simulink model "car_model"  (R2019b)
settings: Solver=ode23tb  StartTime=0.0  StopTime=60  RelTol=1e-3
InitFcn:
  | CommonVariables
  | Klqr5Velocities
values from neighbouring files (symbols this model uses):
  BattChrgMax = -80000    [CommonVariables.m]
  BattDischrgMax = 80000    [CommonVariables.m]
  BrkPrsMax = 5000000    [CommonVariables.m]
  ChrgLmt_bpt = [1 1 1 1 1 1 1 1 0.7 0.35 0]    [CommonVariables.m]
  DischrgLmt_bpt = [0 0.35 0.7 1 1 1 1 1 1 1 1]    [CommonVariables.m]
  disk_abore = 0.05    [CommonVariables.m]
  efficiency_table = [85 85 85 85 85 85 85 85 85 85 85 85 85 85 85;85 85 85 85 85 85 85 85 85 85 85 85 85 85 85;85 85 90 90 90 90 90 90 90 90 88 88 88 88 88;85 85 92 92 92 92 92 92 92 92 92 90 90 90 90;85 85 92 92 93 93 93 93 92 92 92 90 90 90 90;85 85 93 94 94 94 94 94 94 94 94 94 94 94 94;85 85 93 94 94 95 95 95 95 95 95 95 95 95 95;85 85 93 94 94 95 95 95 95 95 95 95 95 95 95;85 85 93 94 95 95 95 95 95 95 95 95 95  ...(+141 chars)    [CommonVariables.m]
  F0z = [2886 2907]    [CommonVariables.m]
  h = 0.134    [CommonVariables.m]
  m = 1200    [Klqr5Velocities.m]
  MotSpd = [0 1000 2000 2728.370453 3000 4000 5000 6000 7000 8000 9000 10000]    [CommonVariables.m]
  MotTrq = [280 280 280 280 254.6479089 190.9859317 152.7887454 127.3239545 109.1348181 95.49296586 84.88263632 76.39437268]    [CommonVariables.m]
  mu_kinetic = 0.35    [CommonVariables.m]
  Ndiff = 7.94    [CommonVariables.m]
  num_pads = 2    [CommonVariables.m]
  RegenBrkCutOff = [0 1]    [CommonVariables.m]
  RegenBrkSpd_bpt = [5 9]    [CommonVariables.m]
  Rm = 0.15    [CommonVariables.m]
  SOC_bpt = [0 10 20 30 40 50 60 70 80 90 100]    [CommonVariables.m]
  T_eff_bp = [0 20 40 60 80 100 120 140 160 180 200 220 240 260 280]    [CommonVariables.m]
  w_eff_bp = [0 1000 2000 2728.370453 3000 4000 5000 6000 7000 8000 9000 10000]    [CommonVariables.m]
undefined symbols (not defined in the file or in its folder): Disabled, DLCXref, DLCYref, Klqr1, Klqr2, Klqr3, Klqr4, Klqr5, Right, VEH
libraries: simulink x8, vehdynlibtire x8, vehdynlibsuspension x7, vehdynlibscenariocommon x5, autolibutils x4, sim3dlib x4, autolibmappedmotor x4, autolibshared x2, sharedtransform x2, vehdynlibviscommon x2, vehdynlibdriver x1, vehdynlibsteering x1
(part 1 of 7)
settings Model: SimulationMode=accelerator  OrderedModelArguments=off  Creator=davide  LastModifiedBy=alelu
settings SolverCC: ZeroCrossAlgorithm=Adaptive  AutoInsertRateTranBlk=on  InsertRTBMode=Never (minimum delay)
settings DebuggingCC: ArtificialAlgebraicLoopMsg=none  ModelReferenceExtraNoncontSigs=none
settings ModelReferenceCC: ModelReferenceMinAlgLoopOccurrences=on  PropagateSignalLabelsOutOfModel=off
settings SFSimCC: CustomCodeUndefinedFunction=UseInterfaceOnly

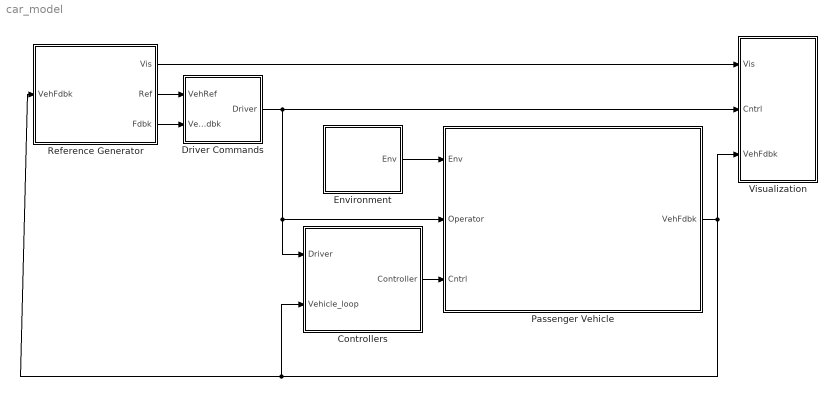
== system car_model ==
  Controllers : Subsystem
      mask Display: image('SystemControllers.png')
  Driver Commands : Subsystem  VariantControl=0  mask{driverType=Predictive Driver}
      mask prompts: driverType "Vehicle command mode"
      mask init:
      | [~]=vdynblksdrvrconfig(gcb)
      settings: AttributesFormatString=%<driverType>
      mask Help: eval('vdynblkshelp(''vdcrdriver'')');
      mask TypeOptions driverType: Longitudinal Driver | Predictive Driver | Open Loop
      mask Display: image('driverlatlong.png');
  Environment : Subsystem
      mask Display: disp('Environment')
  Passenger Vehicle : Subsystem
      mask Display: image('PassengerVehicle.png')
  Reference Generator : Subsystem  mask(Reference Generator){manType=Double Lane Change, manOverride=on, prevType=Double Lane Change, t_start=1, xdot_r=35, xdotUnit=mph, aMode=2, omega_hw=13.5, theta_max=90, t_stop=60, ay_max=.5, ay_stop=on, XGate=174.5, xStart=2, vehW=2, lattoff=VEH.InitialLatPosition, latRefbp=DLCXref, latRef=DLCYref, t_sweep=30, theta_hw=90, theta_hw_final=.7, steerF=.7, steerA=90, tdwell=.5, steerDir=off, R=100, turnDirMask=Right, cr_ay_max=0.5, cr_ay_stop=off, simTime=60, engine3D=Disabled, SceneDesc=Open surface, dt3D=.03, defaultPos=Recommended for scene, X_o=0, Y_o=0, Z_o=0, phi_o=0, theta_o=0, psi_o=0}
      mask prompts: manType "Maneuver"; manOverride "Use maneuver-specific driver, initial position, and scene"; t_start "Maneuver start time, t_start [s]:"; xdot_r "Longitudinal velocity reference, xdot_r:"; xdotUnit "Longitudinal entrance velocity setpoint units, xdotUnit []:"; omega_hw "Handwheel rate, omega_hw [deg/s]:"; theta_max "Maximum handwheel angle, theta_max [deg]:"; t_stop "Steering hold time after max angle reached, t_stop [s]:"; ay_max "Lateral acceleration threshold, ay_max [g]:"; ay_stop "Stop simulation at lateral acceleration threshold"; XGate "Inertial longitudinal position of gate entrance, XGate [m]:"; xStart "Distance after target speed to begin reference, x_start [m]:"; vehW "Vehicle width, vehW [m]:"; lattoff "Lateral offset, latoff [m]:"; latRefbp "Lateral reference position breakpoints [m]:"; latRef "Lateral reference data, latRef [m]:"; t_sweep "Swept time, t_sweep [s]:"; theta_hw "Steering amplitude, theta_hw [deg]"; theta_hw_final "Final frequency, theta_hw_final [Hz]:"; steerF "Steer frequency, steerF [Hz]:"; steerA "Steer amplitude, steerA [deg]:"; tdwell "Dwell time, tdwell [s]:"; steerDir "Change direction, steerDir"; R "Radius value, R [m]:"; turnDirMask "Turn direction"; cr_ay_max "Lateral acceleration threshold, ay_max [g]:"; cr_ay_stop "Stop simulation at lateral acceleration threshold"; simTime "Simulation time, simTime [s]:"; engine3D "3D Engine"; SceneDesc "Scene:"; dt3D "Engine frame rate, dt3D [s]:"; X_o "Initial longitudinal position, X_o [m]:"; Y_o "Initial lateral position, Y_o [m]:"; Z_o "Initial vertical position, Z_o [m]:"; phi_o "Initial roll angle, phi_o [rad]:"; theta_o "Initial pitch angle, theta_o [rad]:"; psi_o "Initial yaw angle, psi_o [rad]:"
      mask help: Set parameters to configure the maneuver, driver model, and 3D environment. To set the initial vehicle position and orientation, use the parameters on the 3D Engine tab.
      mask init:
      | set_param(gcb,'prevType',get_param(gcb,'manType'))
      settings: AttributesFormatString=%<manType>
      mask Help: eval('vdynblkshelp(''vdcrrefgen'')');
      mask TypeOptions manType: Double Lane Change | Increasing Steer | Swept Sine | Sine with Dwell | Constant Radius
      mask Callback manType:
      | [~]=vdynblksrefconfig(gcb,0);
      | [~]=vdynblksrefconfig(gcb,1);
      mask TypeOptions prevType: Double Lane Change | Increasing Steer | Swept Sine | Sine with Dwell | Constant Radius
      mask TypeOptions xdotUnit: Reference Generator/Double Lane Change/Double Lane Change/xdotUnit | Reference Generator/Constant Radius/xdotUnit | Reference Generator/Increasing Steer/Increasing Steer/xdotUnit | Reference Generator/Sine with Dwell/Sine With Dwell/xdotUnit | Reference Generator/Swept Sine/Swept Sine/xdotUnit
      mask TypeOptions omega_hw: Reference Generator/Increasing Steer/Increasing Steer/omega_hw
      mask TypeOptions theta_max: Reference Generator/Increasing Steer/Increasing Steer/theta_max
      mask TypeOptions t_stop: Reference Generator/Increasing Steer/Increasing Steer/t_stop
      mask TypeOptions ay_max: Reference Generator/Increasing Steer/Increasing Steer/ay_max
      mask TypeOptions ay_stop: Reference Generator/Increasing Steer/Increasing Steer/ay_stop
      mask Callback ay_stop:
      | if strcmp(get_param(gcb,'ay_stop'),'off')
      |     autoblksenableparameters(gcb, [], {'ay_max'},[],[],true);
      | else
      |     autoblksenableparameters(gcb,{'ay_max'},[],[],[],true);
      | end
      mask TypeOptions XGate: Reference Generator/Double Lane Change/Double Lane Change/XGate
      mask TypeOptions xStart: Reference Generator/Double Lane Change/Double Lane Change/xStart
      mask TypeOptions vehW: Reference Generator/Double Lane Change/Double Lane Change/vehW
      mask TypeOptions lattoff: Reference Generator/Double Lane Change/Double Lane Change/lattoff
      mask TypeOptions latRefbp: Reference Generator/Double Lane Change/Double Lane Change/latRefbp
      mask TypeOptions latRef: Reference Generator/Double Lane Change/Double Lane Change/latRef
      mask TypeOptions t_sweep: Reference Generator/Swept Sine/Swept Sine/t_sweep
      mask TypeOptions theta_hw: Reference Generator/Swept Sine/Swept Sine/theta_hw
      mask TypeOptions theta_hw_final: Reference Generator/Swept Sine/Swept Sine/theta_hw_final
      mask TypeOptions steerF: Reference Generator/Sine with Dwell/Sine With Dwell/steerF
      mask TypeOptions steerA: Reference Generator/Sine with Dwell/Sine With Dwell/steerA
      mask TypeOptions tdwell: Reference Generator/Sine with Dwell/Sine With Dwell/tdwell
      mask TypeOptions steerDir: Reference Generator/Sine with Dwell/Sine With Dwell/steerDir
      mask TypeOptions R: Reference Generator/Constant Radius/R
      mask TypeOptions turnDirMask: Reference Generator/Constant Radius/turnDirMask
      mask TypeOptions cr_ay_max: Reference Generator/Constant Radius/ay_max
      mask TypeOptions cr_ay_stop: Reference Generator/Constant Radius/ay_stop
      mask Callback cr_ay_stop:
      | if strcmp(get_param(gcb,'cr_ay_stop'),'off')
      |     autoblksenableparameters(gcb, [], {'cr_ay_max'},[],[],true);
      | else
      |     autoblksenableparameters(gcb,{'cr_ay_max'},[],[],[],true);
      | end
      mask TypeOptions engine3D: 3D Engine/engine3D
      mask TypeOptions SceneDesc: 3D Engine/SceneDesc
      mask Callback SceneDesc: [~] = vdynblks3Dsceneconfig(gcb);
      mask TypeOptions dt3D: 3D Engine/dt3D
      mask TypeOptions defaultPos: Recommended for scene | User-specified
      mask TypeOptions X_o: 3D Engine/X_o
      mask TypeOptions Y_o: 3D Engine/Y_o
      mask TypeOptions Z_o: 3D Engine/Z_o
      mask TypeOptions phi_o: 3D Engine/phi_o
      mask TypeOptions theta_o: 3D Engine/theta_o
      mask TypeOptions psi_o: 3D Engine/psi_o
      mask DialogControl modTab Prompt: Model
      mask DialogControl configGroup Prompt: Configuration
      mask DialogControl ISGroup Prompt: Increasing Steer
      mask DialogControl DLCGroup Prompt: Double Lane Change
      mask DialogControl SSGroup Prompt: Swept Sine
      mask DialogControl SDGroup Prompt: Sine with Dwell
      mask DialogControl CRGroup Prompt: Constant Radius
      mask DialogControl simUpdate Prompt: Set Model Simulation Time
      mask DialogControl simUpdate Callback: [~]=vdynblksrefconfig(gcb,2);
      mask DialogControl sim3DTab Prompt: 3D Engine
      mask DialogControl sim3DGroup Prompt: 3D Engine
      mask DialogControl posSetupDesc Prompt: To use these initial vehicle positions, first Apply the initial values and then click Update the model workspaces with the initial values.
      mask DialogControl setModelPos Prompt: Update model workspaces with initial values
      mask DialogControl setModelPos Callback: [~] = vdynblksmdlWSconfig(gcb);
      mask Display: image('vdbslibscen.png')
  Visualization : Subsystem
      mask Display: disp('Visualization')
  wires:
  Passenger Vehicle/1(VehFdbk) -> Controllers/2(Vehicle_loop), Reference Generator/1("VehFdbk "), Visualization/3(VehFdbk)
  Reference Generator/1(" Vis") -> Visualization/1(Vis)
  Reference Generator/2(" Ref") -> Driver Commands/1(VehRef)
  Controllers/1(Controller) -> Passenger Vehicle/3(Cntrl)
  Reference Generator/3(" Fdbk") -> Driver Commands/2(VehFdbk)
  Environment/1(Env) -> Passenger Vehicle/1(Env)
  Driver Commands/1(Driver) -> Passenger Vehicle/2(Operator), Controllers/1(Driver), Visualization/2(Cntrl)

== system car_model/Controllers ==
  Driver : Inport
  Vehicle_loop : Inport  Port=2
  Accel Pedal to Traction Wheel Torque Request : Subsystem
  Battery Management System : Subsystem
  Brake Pedal to Total Braking Pressure Request : Subsystem
  Bus Creator2 : BusCreator  Inputs=1
  Bus Creator3 : BusCreator  Inputs=3
  Bus Selector : BusSelector  OutputSignals=Body.r,Body.xdot,Body.ydot,Driveline.WhlAng,ElecFdbk.BattSoc,Driveline.EngSpd
  Bus Selector3 : BusSelector  OutputSignals=Steer,Accel,Brake
  Constant : Constant  Value=0
  Motor Torque Arbitration and Power Management : Subsystem
  Regen Braking Control : Subsystem  VariantControlMode=Label  Variant=on  VariantControl=(default)  LabelModeActiveChoice=Variant
  Controller : Outport  VectorParamsAs1DForOutWhenUnconnected=off
  wires:
  Driver/1 -> Bus Selector3/1
  Motor Torque Arbitration and Power Management/1(MotTrqCmdFinal) -> Bus Creator3/1  "acc"
  Bus Creator2/1 -> Bus Creator3/2  "Brake"
  Bus Creator3/1 -> Controller/1  "Controller"
  Battery Management System/1(BattPwrDischrgLmt) -> Motor Torque Arbitration and Power Management/3(BattPwrDisChrgLmt)  "BattPwrDischrgLmt"
  Regen Braking Control/1(" MotTrqCmdRegen") -> Motor Torque Arbitration and Power Management/6(MotTrqCmdRegen)  "MotTrqCmdRegen"
  [MotSpd] -> Motor Torque Arbitration and Power Management/5(MotSpd)
  Bus Selector/6 -> Regen Braking Control/2("VehSpd "), [MotSpd], Regen Braking Control/3("MotSpd ")  "<EngSpd>"
  Accel Pedal to Traction Wheel Torque Request/1(TrqCmd) -> Motor Torque Arbitration and Power Management/1(MotTrqCmdTrac)
  Battery Management System/2(BattPwrChrgLmt) -> Motor Torque Arbitration and Power Management/4("BattPwrChrgLmt ")  "BattPwrChrgLmt"
  Bus Selector3/3 -> Brake Pedal to Total Braking Pressure Request/1(DecelPdl)  "<Brake>"
  Regen Braking Control/2(" BrkCmd") -> Bus Creator2/1  "BrkCmd"
  Constant/1 -> Brake Pedal to Total Braking Pressure Request/2(Park)
  [MotSpd] -> Accel Pedal to Traction Wheel Torque Request/6(MotSpd)
  Bus Selector/5 -> Battery Management System/1(SOC), Regen Braking Control/1("BattSoc ")  "<BattSoc>"
  Brake Pedal to Total Braking Pressure Request/1(BrkPrsReq) -> Regen Braking Control/4("BrkPrsReq ")
  [AccelPdl] -> Motor Torque Arbitration and Power Management/2(AccelPdl)
  Bus Selector3/2 -> Accel Pedal to Traction Wheel Torque Request/1(AccelPdl), [AccelPdl]  "<Accel>"
  Vehicle_loop/1 -> Bus Selector/1
  Bus Selector/4 -> Accel Pedal to Traction Wheel Torque Request/2(WhlAng)  "<WhlAng>"
  Bus Selector/1 -> Accel Pedal to Traction Wheel Torque Request/5(YawRate)  "<r>"
  Bus Selector/2 -> Accel Pedal to Traction Wheel Torque Request/3(xdot)  "<xdot>"
  Bus Selector/3 -> Accel Pedal to Traction Wheel Torque Request/4(ydot)  "<ydot>"

== system car_model/Driver Commands ==
  VehRef : Inport
  VehFdbk : Inport  Port=2
  AccelGround : Ground
  BrakeGround : Ground
  Driver Commands : Subsystem  VariantControlMode=Label  Variant=on  VariantControl=Variant1  LabelModeActiveChoice=1  AllowZeroVariantControls=on
  GearGround : Ground
  SteerGround : Ground
  Driver : Outport  VectorParamsAs1DForOutWhenUnconnected=off
  wires:
  VehRef/1 -> Driver Commands/1(VehRef)
  VehFdbk/1 -> Driver Commands/2(VehFdbk)
  Driver Commands/1(" Driver") -> Driver/1
  SteerGround/1 -> Driver Commands/3(SteerCmd)
  AccelGround/1 -> Driver Commands/4(Accel)
  BrakeGround/1 -> Driver Commands/5(Brake)
  GearGround/1 -> Driver Commands/6(Gear)

== system car_model/Environment ==
  Bus Creator1 : BusCreator  Inputs=4
  Constant3 : Constant  Value=0
  Constant4 : Constant  Value=0
  Constant5 : Constant  Value=0
  Constant6 : Constant  Value=300
  Constant7 : Constant  Value=101325
  Friction : Constant  Value=ones(4,1).*1
  Ground Feedback : Subsystem  VariantControlMode=Label  Variant=on  LabelModeActiveChoice=0
  Vector Concatenate : Concatenate  NumInputs=3
  Env : Outport  VectorParamsAs1DForOutWhenUnconnected=off
  wires:
  Constant5/1 -> Vector Concatenate/3  "Z"
  Vector Concatenate/1 -> Bus Creator1/3  "Wind"
  Constant3/1 -> Vector Concatenate/1  "X"
  Constant4/1 -> Vector Concatenate/2  "Y"
  Ground Feedback/1(Ground) -> Bus Creator1/4  "Gnd"
  Bus Creator1/1 -> Env/1
  Friction/1 -> Ground Feedback/1(Friction)
  Constant6/1 -> Bus Creator1/1  "Temp"
  Constant7/1 -> Bus Creator1/2  "Baro"

== system car_model/Passenger Vehicle ==
  Env : Inport
  Operator : Inport  Port=2
  Cntrl : Inport  Port=3
  Bus Creator2 : BusCreator  Inputs=4
  Subsystem : Subsystem
  Subsystem1 : Subsystem
  Subsystem2 : Subsystem
  Subsystem4 : Subsystem
  Subsystem5 : Subsystem
  Subsystem6 : Subsystem
  VehFdbk : Outport  VectorParamsAs1DForOutWhenUnconnected=off
  wires:
  Bus Creator2/1 -> VehFdbk/1
  Env/1 -> Subsystem2/4(Env), Subsystem/1(Env)
  Subsystem1/1(Driveline) -> [Driveline], Bus Creator2/1  "Driveline"
  Subsystem5/1(WhlAng) -> Subsystem1/1(WhlAng)
  Operator/1 -> Subsystem2/2(SteerCmd)
  Cntrl/1 -> Subsystem2/1(Cntrl)
  Subsystem2/1(Steer) -> Subsystem5/1(SteerHWCmd)
  Subsystem2/2(brake) -> Subsystem5/2(BrkPrsCmd)
  Subsystem4/2(Wheels) -> Bus Creator2/4, [Wheels]  "Wheels"
  [Driveline] -> Subsystem/2(Driveline)
  [Wheels] -> Subsystem2/3(Wheels)
  Subsystem6/15(dzWheel) -> Subsystem4/15(dzWheel)
  Subsystem6/3(CgXYZdot) -> Subsystem4/3(CgXYZdot)
  Subsystem6/1(Cgxyzdot) -> Subsystem4/1(Cgxyzdot)
  Subsystem6/5(pqr) -> Subsystem4/5(pqr)
  Subsystem6/14(YWheel) -> Subsystem4/14(YWheel)
  Subsystem6/7(Beta) -> Subsystem4/7(Beta)
  Subsystem6/6(Cgaxyz) -> Subsystem4/6(Cgaxyz)
  Subsystem6/8(GeomXYZ) -> Subsystem4/8(GeomXYZ)
  Subsystem6/4(angles) -> Subsystem4/4(angles)
  Subsystem6/11(kappa) -> Subsystem4/11(kappa)
  Subsystem6/13(XWheel) -> Subsystem4/13(XWheel)
  Subsystem6/2(CgXYZ) -> Subsystem4/2(CgXYZ)
  Subsystem6/9(GeomXYZdot) -> Subsystem4/9(GeomXYZdot)
  Subsystem6/10(omega) -> Subsystem4/10(omega)
  Subsystem6/12(alpha) -> Subsystem4/12(alpha)
  Subsystem5/2(BrkPrs) -> Subsystem1/2(BrkPrs)
  Subsystem5/5(BattSoc) -> Subsystem1/5(BattSoc)
  Subsystem5/6(BattPwr) -> Subsystem1/6(BattPwr)
  Subsystem5/7(BattCrnt) -> Subsystem1/7(BattCrnt)
  Subsystem2/4(acc) -> Subsystem5/4("acc ")
  Subsystem5/3(AxlTrq) -> Subsystem1/3(AxlTrq)
  Subsystem5/4(Motor_speed) -> Subsystem1/4(EngSpd)
  Subsystem2/5(amb_temp) -> Subsystem5/5(AmbTmp)
  Subsystem2/3(omega) -> Subsystem5/3(speed_wheel)
  Subsystem1/2(ElecFdbk) -> Bus Creator2/2  "ElecFdbk"
  Subsystem4/1(Chassis) -> Bus Creator2/3  "Body"
  Subsystem/1(Wind) -> Subsystem6/1(WindXYZ)
  Subsystem/2(Gnd) -> Subsystem6/2(Ground)
  Subsystem/3(mu) -> Subsystem6/3(Friction)
  Subsystem/4(WhlAng) -> Subsystem6/4(WheelAngle)
  Subsystem/5(AxleTrq) -> Subsystem6/5(AxleTrq)
  Subsystem/6(BrkPrs) -> Subsystem6/6(BrkPrs)

== system car_model/Reference Generator ==
  "VehFdbk " : Inport
  3D Engine : Subsystem  VariantControlMode=Label  Variant=on  LabelModeActiveChoice=0  mask(3D Engine){engine3D=Disabled, SceneDesc=Open surface, dt3D=dt3D, defaultPos=User-specified, X_o=X_o, Y_o=Y_o, Z_o=Z_o, phi_o=phi_o, theta_o=theta_o, psi_o=psi_o}
      mask prompts: engine3D "3D Engine"; SceneDesc "Scene:"; dt3D "Engine frame rate, dt3D [s]:"; X_o "Initial longitudinal position, X_o [m]:"; Y_o "Initial lateral position, Y_o [m]:"; Z_o "Initial vertical position, Z_o [m]:"; phi_o "Initial roll angle, phi_o [rad]:"; theta_o "Initial pitch angle, theta_o [rad]:"; psi_o "Initial yaw angle, psi_o [rad]:"
      mask help: This subsystem contains the interface blocks which permit the display of the vehicle in the 3D virtual environment. Enable it to view the simulation progress, disable it to inhibit the display.
      mask init:
      | switch get_param(gcb,'engine3D')
      |     case 'Disabled'
      |         set_param(gcb,'OverrideUsingVariant','0')
      |         try
      |             set_param([bdroot '/Environment/Ground Feedback'],'OverrideUsingVariant','0')
      |         catch
      |             disp('Warning: No ground feedback sensor not set')
      |         end
      |     case 'Enabled'
      |         set_param(gcb,'OverrideUsingVariant','1')
      |         try
      |             set_param([bdroot '/Environment/Ground Feedback'],'OverrideUsingVariant','1')
      |         catch
      |             disp('Warning: No ground feedback sensor not set')
      |         end
      |     otherwise
      |         set_param(gcb,'OverrideUsingVariant','0')
      | end
      settings: AttributesFormatString=|
      | %<SceneDesc>
      | %<engine3D>
      mask Help: eval('vdynblkshelp(''vdynblks3dengine'')');
      mask TypeOptions engine3D: Enabled | Disabled
      mask Callback engine3D:
      | switch get_param(gcb,'engine3D')
      |     case 'Disabled'
      |         set_param(gcb,'OverrideUsingVariant','0')
      |     case 'Enabled'
      |        set_param(gcb,'OverrideUsingVariant','1')
      |     otherwise
      |        set_param(gcb,'OverrideUsingVariant','0')
      | end
      mask TypeOptions SceneDesc:
      | 3D Engine/Simulation 3D Engine
      | 1/SceneDesc
      mask Callback SceneDesc: [~] = vdynblks3Dsceneconfig(gcb);
      mask TypeOptions defaultPos: Recommended for scene | User-specified
      mask DialogControl engineConfig Prompt: 3D Engine Settings
      mask DialogControl posSetup Prompt: Initial vehicle position
      mask DialogControl posSetupDesc Prompt: To use these initial vehicle positions, first Apply the initial values and then click Update the model workspaces with the initial values.
      mask DialogControl setModelPos Prompt: Update model workspaces with initial values
      mask DialogControl setModelPos Callback: [~] = vdynblksmdlWSconfig(gcb);
      mask Display: disp('3D Engine')
  Reference Generator : Subsystem  VariantControlMode=Label  Variant=on  VariantControl=Variant1  LabelModeActiveChoice=4
  " Vis" : Outport  VectorParamsAs1DForOutWhenUnconnected=off
  " Ref" : Outport  Port=2  VectorParamsAs1DForOutWhenUnconnected=off
  " Fdbk" : Outport  Port=3  VectorParamsAs1DForOutWhenUnconnected=off
  wires:
  "VehFdbk "/1 -> 3D Engine/1(VehFdbk), Reference Generator/1("VehFdbk ")
  Reference Generator/1(" Vis") -> " Vis"/1
  Reference Generator/2(" Ref") -> " Ref"/1
  Reference Generator/3(" Fdbk") -> " Fdbk"/1

== system car_model/Visualization ==
  note: Vehicle Response
  note: Driver Commands
  Vis : Inport
  Cntrl : Inport  Port=2
  VehFdbk : Inport  Port=3
  Acceleration Cmd : LinearGaugeBlock  LabelPosition=Hide  ScaleMax=1  TickInterval=0.20000000000000001
  Brake Cmd : LinearGaugeBlock  LabelPosition=Hide  ScaleMax=1  TickInterval=0.20000000000000001
  Bus Selector : BusSelector  OutputSignals=Body.xdot,Body.ay
  Bus Selector2 : BusSelector  OutputSignals=Accel,Brake,Steer
  Engine Tach [rpm] : CircularGaugeBlock  LabelPosition=Hide  ScaleMax=8000  TickInterval=1000
  Handwheel Angle [deg] : SemiCircularGaugeBlock  LabelPosition=Hide  ScaleMin=-300  ScaleMax=300  TickInterval=60
  ISO 15037-1:2006 : Subsystem  StopFcn=|  VariantControlMode=Label  Variant=on  LabelModeActiveChoice=0  mask(ISO 15037-1:2006){Measurement=Disabled}
      | switch get_param(gcb,'Measurement')
      |     case 'Enabled'
      |        p=slproject.getCurrentProject;
      |        projectRoot=p.RootFolder;
      |        SySFolder=fullfile(projectRoot, 'System');
      |        Simulink.sdi.loadView([SySFolder filesep 'ISO15037_1_2006E.mldatx']);
      |        Simulink.sdi.view;
      | end
      mask prompts: Measurement "ISO Measurements"
      mask help: Enables display of ISO 15037-1:2006 standard measurement signals in the Simulation Data Inspector.
      mask init:
      | switch get_param(gcb,'Measurement')
      |     case 'Disabled'
      |         set_param(gcb,'OverrideUsingVariant','0')
      |     case 'Enabled'
      |        set_param(gcb,'OverrideUsingVariant','1')
      |     otherwise
      |        set_param(gcb,'OverrideUsingVariant','0')
      | end
      settings: AttributesFormatString=%<Measurement>
      mask Help: eval('vdynblkshelp(''iso15037'')');
      mask TypeOptions Measurement: Enabled | Disabled
      mask Callback Measurement:
      | switch get_param(gcb,'Measurement')
      |     case 'Disabled'
      |         set_param(gcb,'OverrideUsingVariant','0')
      |     case 'Enabled'
      |        set_param(gcb,'OverrideUsingVariant','1')
      |     otherwise
      |        set_param(gcb,'OverrideUsingVariant','0')
      | end
      mask Display: disp('ISO 15037-1:2006')
  Lateral Acceleration [g] : SemiCircularGaugeBlock  LabelPosition=Hide  ScaleMin=-1  ScaleMax=1  TickInterval=0.5
  Rate Transition1 : RateTransition  Deterministic=off  OutPortSampleTime=.1
  Rate Transition2 : RateTransition  Deterministic=off  OutPortSampleTime=.1
  Scope Type : Subsystem  VariantControlMode=Label  Variant=on  VariantControl=Variant1  LabelModeActiveChoice=2
  Signal Specification : SignalSpecification  Unit=deg
  Signal Specification1 : SignalSpecification  Unit=mph
  Speed [mph] : CircularGaugeBlock  LabelPosition=Hide  TickInterval=10
  Steer vs Ay : simulink/Sinks/XY Graph  Commented=on  xmin=-300  xmax=300  ymin=-1.5  ymax=1.5  st=.1
  "Steer, Velocity, Lat Accel" : Scope  NumInputPorts=3
  Terminator : Terminator
  Terminator1 : Terminator
  Terminator2 : Terminator
  Unit Conversion1 : UnitConversion
  Unit Conversion2 : UnitConversion
  Vehicle XY Plotter : Subsystem  VariantControlMode=Label  Variant=on  VariantControl=Variant1  LabelModeActiveChoice=1
  wires:
  Signal Specification/1 -> Rate Transition1/1, "Steer, Velocity, Lat Accel"/1  "SteerAngle"
  Bus Selector/2 -> "Steer, Velocity, Lat Accel"/3, Rate Transition2/1  "<ay>"
  Bus Selector/1 -> "Steer, Velocity, Lat Accel"/2, Unit Conversion1/1  "<xdot>"
  Unit Conversion2/1 -> Signal Specification/1
  Unit Conversion1/1 -> Signal Specification1/1
  Signal Specification1/1 -> Terminator/1  "xdot_mph"
  Bus Selector2/3 -> Unit Conversion2/1  "<Steer>"
  Rate Transition1/1 -> Steer vs Ay/1
  Rate Transition2/1 -> Steer vs Ay/2
  Bus Selector2/1 -> Terminator1/1  "<Accel>"
  Bus Selector2/2 -> Terminator2/1  "<Brake>"
  VehFdbk/1 -> ISO 15037-1:2006/1(VehFdbk), Scope Type/1("VehFdbk "), Vehicle XY Plotter/1("VehFdbk "), Bus Selector/1  "VehFdbk"
  Cntrl/1 -> ISO 15037-1:2006/2(Cntrl), Scope Type/2(Cntrl), Bus Selector2/1
  Vis/1 -> Scope Type/3("Vis ")
  Scope Type/1(" Ref") -> Vehicle XY Plotter/2("Ref ")

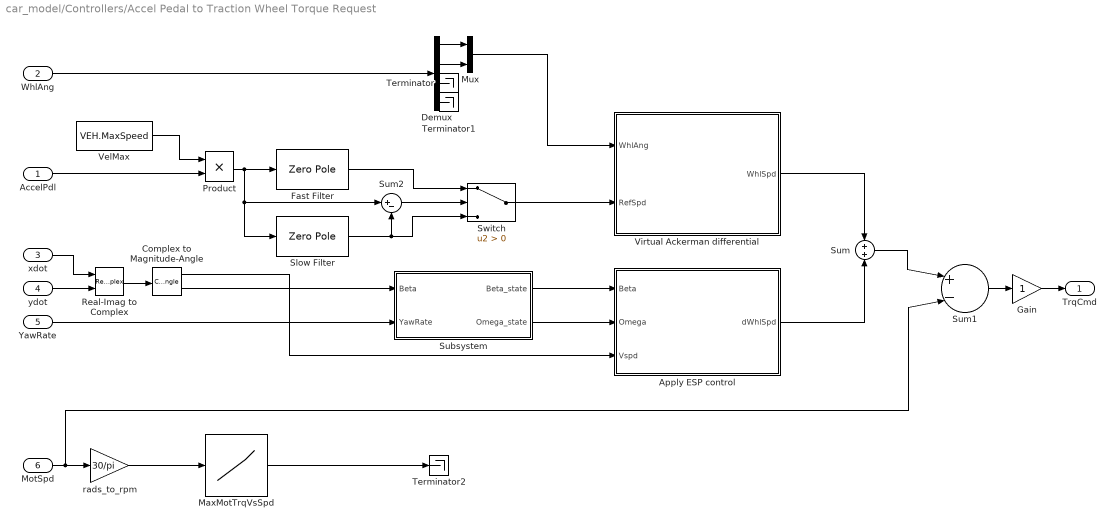
== system car_model/Controllers/Accel Pedal to Traction Wheel Torque Request ==
  AccelPdl : Inport
  WhlAng : Inport  Port=2
  xdot : Inport  Port=3
  ydot : Inport  Port=4
  YawRate : Inport  Port=5
  MotSpd : Inport  Port=6
  Apply ESP control : Subsystem
  Complex to Magnitude-Angle : ComplexToMagnitudeAngle
  Demux : Demux
  Fast Filter : ZeroPole  Zeros=[]  Poles=[-20]
  Gain : Gain
  MaxMotTrqVsSpd : Lookup_n-D  NumberOfTableDimensions=1  BreakpointsForDimension1=MotSpd  Table=MotTrq  ExtrapMethod=Clip  UseLastTableValue=on  InternalRulePriority=Speed  OutDataTypeStr=Inherit: Inherit from 'Table data'  RndMeth=Simplest  InputSameDT=on
  Mux : Mux  Inputs=2
  Product : Product
  Real-Imag to Complex : RealImagToComplex
  Slow Filter : ZeroPole  Zeros=[]  Poles=[-2]
  Subsystem : Subsystem
  Sum : Sum  Inputs=+|+
  Sum1 : Sum  Inputs=|+-|
  Sum2 : Sum  Inputs=|+-
  Switch : Switch  Criteria=u2 > Threshold
  Terminator : Terminator
  Terminator1 : Terminator
  Terminator2 : Terminator
  VelMax : Constant  Value=VEH.MaxSpeed
  Virtual Ackerman differential : Subsystem
  rads_to_rpm : Gain  Gain=30/pi
  TrqCmd : Outport  VectorParamsAs1DForOutWhenUnconnected=off
  wires:
  MaxMotTrqVsSpd/1 -> Terminator2/1
  MotSpd/1 -> Sum1/2, rads_to_rpm/1
  rads_to_rpm/1 -> MaxMotTrqVsSpd/1
  Subsystem/1(Beta_state) -> Apply ESP control/1(Beta)
  Subsystem/2(Omega_state) -> Apply ESP control/2(Omega)
  Real-Imag to Complex/1 -> Complex to Magnitude-Angle/1
  xdot/1 -> Real-Imag to Complex/1
  ydot/1 -> Real-Imag to Complex/2
  Complex to Magnitude-Angle/1 -> Apply ESP control/3(Vspd)
  Complex to Magnitude-Angle/2 -> Subsystem/1(Beta)
  YawRate/1 -> Subsystem/2(YawRate)
  Virtual Ackerman differential/1(WhlSpd) -> Sum/1
  Apply ESP control/1(dWhlSpd) -> Sum/2
  Sum/1 -> Sum1/1
  VelMax/1 -> Product/1
  AccelPdl/1 -> Product/2
  Product/1 -> Fast Filter/1, Slow Filter/1, Sum2/1
  Fast Filter/1 -> Switch/1
  Sum1/1 -> Gain/1
  Gain/1 -> TrqCmd/1
  Demux/1 -> Mux/1
  Demux/2 -> Mux/2
  WhlAng/1 -> Demux/1
  Mux/1 -> Virtual Ackerman differential/1(WhlAng)
  Sum2/1 -> Switch/2
  Slow Filter/1 -> Switch/3, Sum2/2
  Switch/1 -> Virtual Ackerman differential/2(RefSpd)

== system car_model/Controllers/Battery Management System ==
  note: Behaviorial BMS System. Limits battery charge / discharge power based on SOC.
      |
      | Charge/Discharge Limits and curves can be adjusted if using a larger battery pack
      | or motor power is changed.
  SOC : Inport
  ChrgLmt : Lookup_n-D  NumberOfTableDimensions=1  BreakpointsForDimension1=SOC_bpt  Table=ChrgLmt_bpt  ExtrapMethod=Clip  UseLastTableValue=on  InternalRulePriority=Speed  RndMeth=Simplest  InputSameDT=on
  DischrgLmt : Lookup_n-D  NumberOfTableDimensions=1  BreakpointsForDimension1=SOC_bpt  Table=DischrgLmt_bpt  ExtrapMethod=Clip  UseLastTableValue=on  InternalRulePriority=Speed  RndMeth=Simplest  InputSameDT=on
  MaxChrg : Constant  Value=BattChrgMax
  MaxDischrg : Constant  Value=BattDischrgMax
  Product : Product
  Product1 : Product
  BattPwrDischrgLmt : Outport  VectorParamsAs1DForOutWhenUnconnected=off
  BattPwrChrgLmt : Outport  Port=2  VectorParamsAs1DForOutWhenUnconnected=off
  wires:
  SOC/1 -> DischrgLmt/1, ChrgLmt/1
  MaxChrg/1 -> Product1/2
  MaxDischrg/1 -> Product/2
  Product/1 -> BattPwrDischrgLmt/1
  Product1/1 -> BattPwrChrgLmt/1
  ChrgLmt/1 -> Product1/1
  DischrgLmt/1 -> Product/1

== system car_model/Controllers/Brake Pedal to Total Braking Pressure Request ==
  note: Converts Brake Pedal Position to Brake Pressure Request
  DecelPdl : Inport
  Park : Inport  Port=2
  Constant : Constant  Value=BrkPrsMax
  Constant1 : Constant
  Product1 : Product
  Switch : Switch  Criteria=u2 > Threshold
  BrkPrsReq : Outport  VectorParamsAs1DForOutWhenUnconnected=off
  wires:
  Constant/1 -> Product1/2
  Switch/1 -> Product1/1
  DecelPdl/1 -> Switch/3
  Constant1/1 -> Switch/1
  Product1/1 -> BrkPrsReq/1
  Park/1 -> Switch/2

== system car_model/Controllers/Motor Torque Arbitration and Power Management ==
  MotTrqCmdTrac : Inport
  AccelPdl : Inport  Port=2
  BattPwrDisChrgLmt : Inport  Port=3
  "BattPwrChrgLmt " : Inport  Port=4
  MotSpd : Inport  Port=5
  MotTrqCmdRegen : Inport  Port=6
  Accel Decel Switch : Switch  Criteria=u2 > Threshold
  Compare To Constant : simulink/Logic and Bit Operations/Compare To Constant  relop=>  const=0  OutDataTypeStr=boolean
  Power Management : Subsystem
  MotTrqCmdFinal : Outport  VectorParamsAs1DForOutWhenUnconnected=off
  wires:
  AccelPdl/1 -> Compare To Constant/1
  MotTrqCmdRegen/1 -> Accel Decel Switch/3
  MotTrqCmdTrac/1 -> Accel Decel Switch/1
  Power Management/1(MotTrqCmdFinal) -> MotTrqCmdFinal/1
  Accel Decel Switch/1 -> Power Management/4(MotTrqCmd)
  BattPwrDisChrgLmt/1 -> Power Management/1(BattPwrDischrgLmt)
  "BattPwrChrgLmt "/1 -> Power Management/2(BattPwrChrgLmt)
  MotSpd/1 -> Power Management/3(MotSpd)
  Compare To Constant/1 -> Accel Decel Switch/2

== system car_model/Controllers/Regen Braking Control ==
  "BattSoc " : Inport
  "VehSpd " : Inport  Port=2
  "MotSpd " : Inport  Port=3
  "BrkPrsReq " : Inport  Port=4
  Parallel Regen Braking : Subsystem  InitFcn=%[~]=autosharedicon('autolibutils',gcb,0);  VariantControl=(default)
  Series Regen Braking : Subsystem  InitFcn=%[~]=autosharedicon('autolibutils',gcb,0);  VariantControl=Variant
  " MotTrqCmdRegen" : Outport  VectorParamsAs1DForOutWhenUnconnected=off
  " BrkCmd" : Outport  Port=2  VectorParamsAs1DForOutWhenUnconnected=off

== system car_model/Driver Commands/Driver Commands ==
  VehRef : Inport
  VehFdbk : Inport  Port=2
  SteerCmd : Inport  Port=3
  Accel : Inport  Port=4
  Brake : Inport  Port=5
  Gear : Inport  Port=6
  Longitudinal Driver : Subsystem  VariantControl=0
  Open Loop Constant Radius : Subsystem  VariantControl=2
  Predictive Driver : Subsystem  VariantControl=1
  " Driver" : Outport  VectorParamsAs1DForOutWhenUnconnected=off

== system car_model/Environment/Ground Feedback ==
  note: 1) Add Subsystem or Model blocks as valid variant choices.
      | 2) You cannot connect blocks at this level. At simulation, connectivity is automatically
      | determined, based on the active variant and port name matching.
  Friction : Inport
  3D Engine : Subsystem  VariantControl=1
  Constant : Subsystem  VariantControl=0
  Ground : Outport  VectorParamsAs1DForOutWhenUnconnected=off

== system car_model/Passenger Vehicle/Subsystem ==
  Env : Inport
  Driveline : Inport  Port=2
  Bus Selector1 : BusSelector  OutputSignals=Gnd.z.G_FL_z,Gnd.z.G_FR_z,Gnd.z.G_RL_z,Gnd.z.G_RR_z
  Bus Selector2 : BusSelector  OutputSignals=Wind
  Bus Selector3 : BusSelector  OutputSignals=Gnd.mu.mu_FL,Gnd.mu.mu_FR,Gnd.mu.mu_RL,Gnd.mu.mu_RR
  Bus Selector4 : BusSelector  OutputSignals=WhlAng,AxlTrq,BrkPrs
  Vector Concatenate : Concatenate  NumInputs=4
  Vector Concatenate1 : Concatenate  NumInputs=4
  Wind : Outport  VectorParamsAs1DForOutWhenUnconnected=off
  Gnd : Outport  Port=2  VectorParamsAs1DForOutWhenUnconnected=off
  mu : Outport  Port=3  VectorParamsAs1DForOutWhenUnconnected=off
  WhlAng : Outport  Port=4  VectorParamsAs1DForOutWhenUnconnected=off
  AxleTrq : Outport  Port=5  VectorParamsAs1DForOutWhenUnconnected=off
  BrkPrs : Outport  Port=6  VectorParamsAs1DForOutWhenUnconnected=off
  wires:
  Env/1 -> Bus Selector3/1, Bus Selector1/1, Bus Selector2/1
  Bus Selector2/1 -> Wind/1  "<Wind>"
  Bus Selector3/1 -> Vector Concatenate/1  "<mu_FL>"
  Bus Selector3/2 -> Vector Concatenate/2  "<mu_FR>"
  Bus Selector3/3 -> Vector Concatenate/3  "<mu_RL>"
  Bus Selector3/4 -> Vector Concatenate/4  "<mu_RR>"
  Vector Concatenate/1 -> mu/1
  Bus Selector1/1 -> Vector Concatenate1/1  "<G_FL_z>"
  Bus Selector1/2 -> Vector Concatenate1/2  "<G_FR_z>"
  Bus Selector1/3 -> Vector Concatenate1/3  "<G_RL_z>"
  Bus Selector1/4 -> Vector Concatenate1/4  "<G_RR_z>"
  Vector Concatenate1/1 -> Gnd/1
  Driveline/1 -> Bus Selector4/1
  Bus Selector4/2 -> AxleTrq/1  "<AxlTrq>"
  Bus Selector4/1 -> WhlAng/1  "<WhlAng>"
  Bus Selector4/3 -> BrkPrs/1  "<BrkPrs>"

== system car_model/Passenger Vehicle/Subsystem1 ==
  WhlAng : Inport
  BrkPrs : Inport  Port=2
  AxlTrq : Inport  Port=3
  EngSpd : Inport  Port=4
  BattSoc : Inport  Port=5
  BattPwr : Inport  Port=6
  BattCrnt : Inport  Port=7
  Bus Creator1 : BusCreator  Inputs=4
  Bus Creator3 : BusCreator  Inputs=4
  Driveline : Outport  VectorParamsAs1DForOutWhenUnconnected=off
  ElecFdbk : Outport  Port=2  VectorParamsAs1DForOutWhenUnconnected=off
  wires:
  Bus Creator1/1 -> Driveline/1  "Driveline"
  AxlTrq/1 -> Bus Creator1/2, Bus Creator3/4  "AxlTrq"
  WhlAng/1 -> Bus Creator1/1  "WhlAng"
  EngSpd/1 -> Bus Creator1/4  "EngSpd"
  BrkPrs/1 -> Bus Creator1/3  "BrkPrs"
  BattCrnt/1 -> Bus Creator3/3
  BattPwr/1 -> Bus Creator3/2
  BattSoc/1 -> Bus Creator3/1
  Bus Creator3/1 -> ElecFdbk/1  "ElecFdbk"

== system car_model/Passenger Vehicle/Subsystem2 ==
  Cntrl : Inport
  SteerCmd : Inport  Port=2
  Wheels : Inport  Port=3
  Env : Inport  Port=4
  Bus Selector1 : BusSelector  OutputSignals=Steer
  Bus Selector2 : BusSelector  OutputSignals=omega
  Bus Selector3 : BusSelector  OutputSignals=Brake,acc
  Bus Selector4 : BusSelector  OutputSignals=Temp
  Steer : Outport  VectorParamsAs1DForOutWhenUnconnected=off
  brake : Outport  Port=2  VectorParamsAs1DForOutWhenUnconnected=off
  omega : Outport  Port=3  VectorParamsAs1DForOutWhenUnconnected=off
  acc : Outport  Port=4  VectorParamsAs1DForOutWhenUnconnected=off
  amb_temp : Outport  Port=5  VectorParamsAs1DForOutWhenUnconnected=off
  wires:
  Cntrl/1 -> Bus Selector3/1
  SteerCmd/1 -> Bus Selector1/1
  Wheels/1 -> Bus Selector2/1
  Bus Selector2/1 -> omega/1  "<omega>"
  Bus Selector3/1 -> brake/1  "<Brake>"
  Bus Selector1/1 -> Steer/1  "<Steer>"
  Bus Selector3/2 -> acc/1  "<acc>"
  Bus Selector4/1 -> amb_temp/1  "<Temp>"
  Env/1 -> Bus Selector4/1

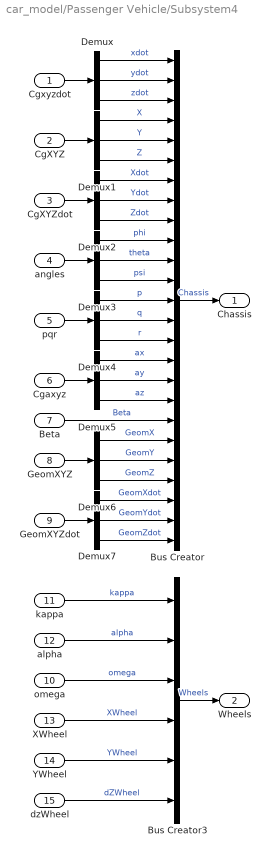
== system car_model/Passenger Vehicle/Subsystem4 ==
  Cgxyzdot : Inport
  CgXYZ : Inport  Port=2
  CgXYZdot : Inport  Port=3
  angles : Inport  Port=4
  pqr : Inport  Port=5
  Cgaxyz : Inport  Port=6
  Beta : Inport  Port=7
  GeomXYZ : Inport  Port=8
  GeomXYZdot : Inport  Port=9
  omega : Inport  Port=10
  kappa : Inport  Port=11
  alpha : Inport  Port=12
  XWheel : Inport  Port=13
  YWheel : Inport  Port=14
  dzWheel : Inport  Port=15
  Bus Creator : BusCreator  Inputs=25
  Bus Creator3 : BusCreator  Inputs=6
  Demux{,1..7} (8 alike) : Demux  Outputs=3
  Chassis : Outport  VectorParamsAs1DForOutWhenUnconnected=off
  Wheels : Outport  Port=2  VectorParamsAs1DForOutWhenUnconnected=off
  wires:
  Bus Creator/1 -> Chassis/1  "Chassis"
  omega/1 -> Bus Creator3/3  "omega"
  dzWheel/1 -> Bus Creator3/6  "dZWheel"
  kappa/1 -> Bus Creator3/1  "kappa"
  Bus Creator3/1 -> Wheels/1  "Wheels"
  YWheel/1 -> Bus Creator3/5  "YWheel"
  XWheel/1 -> Bus Creator3/4  "XWheel"
  alpha/1 -> Bus Creator3/2  "alpha"
  Cgxyzdot/1 -> Demux/1
  CgXYZ/1 -> Demux1/1
  CgXYZdot/1 -> Demux2/1
  angles/1 -> Demux3/1
  pqr/1 -> Demux4/1
  Cgaxyz/1 -> Demux5/1
  GeomXYZdot/1 -> Demux7/1
  GeomXYZ/1 -> Demux6/1
  Demux/1 -> Bus Creator/1  "xdot"
  Demux/2 -> Bus Creator/2  "ydot"
  Demux/3 -> Bus Creator/3  "zdot"
  Demux1/1 -> Bus Creator/4  "X"
  Demux1/2 -> Bus Creator/5  "Y"
  Demux1/3 -> Bus Creator/6  "Z"
  Demux2/1 -> Bus Creator/7  "Xdot"
  Demux2/2 -> Bus Creator/8  "Ydot"
  Demux2/3 -> Bus Creator/9  "Zdot"
  Demux3/1 -> Bus Creator/10  "phi"
  Demux3/2 -> Bus Creator/11  "theta"
  Demux3/3 -> Bus Creator/12  "psi"
  Demux4/1 -> Bus Creator/13  "p"
  Demux4/2 -> Bus Creator/14  "q"
  Demux4/3 -> Bus Creator/15  "r"
  Demux5/1 -> Bus Creator/16  "ax"
  Demux5/2 -> Bus Creator/17  "ay"
  Demux5/3 -> Bus Creator/18  "az"
  Beta/1 -> Bus Creator/19  "Beta"
  Demux6/1 -> Bus Creator/20  "GeomX"
  Demux6/2 -> Bus Creator/21  "GeomY"
  Demux6/3 -> Bus Creator/22  "GeomZ"
  Demux7/1 -> Bus Creator/23  "GeomXdot"
  Demux7/2 -> Bus Creator/24  "GeomYdot"
  Demux7/3 -> Bus Creator/25  "GeomZdot"
